simulink model "GesamtsystemAltV2"  (R2018b)
settings: Solver=FixedStepDiscrete  StartTime=0.0  StopTime=1  RelTol=1e-3  EnableMultiTasking=on
libraries: commutil2 x12, c2833xlib x10, c280xlib x8, powerlib_extras x2, simulink x1, c2000lib x1, dspstat3 x1
(part 3 of 3)

== stateflow chart GesamtsystemAltV2/Subsystem/Sortieralgorithmus2 ==
  state setupVariable
    magacin0 = 0;
    magacin1 = 0;
    magacin2 = 0;
    magacin3 = 0;
    magacin4 = 0;
    magacin5 = 0;
    magacin6 = 0;
    magacin0_LastCube = 0;
    magacin1_LastCube = 0;
    magacin2_LastCube = 0;
    magacin3_LastCube = 0;
    magacin4_LastCube = 0;
    magacin5_LastCube = 0;
    magacin6_LastCube = 0;
    magacin = -1;
    cubeCounter = 0;
    blue = 0;
  state wait
  state cubeLoaded
    magacin = -1
  state photoelectricBarrierActivated
  state BlueCube
    entry: blue = blue + 1;
    entry: magacin = findPlaceForBlue();
  state RedCube
    entry: magacin = findPlaceForRed();
  state Black
    magacin = 6;
    entry: magacin6 = magacin6 + 1;
  state DetectedCube
    entry: cubeCounter = cubeCounter +  1;
  setupVariable -> wait : [switchA > 0]
  (default) -> setupVariable
  wait -> cubeLoaded : [after(2,sec)]
  DetectedCube -> cubeLoaded : [movingCube == 0]
  cubeLoaded -> photoelectricBarrierActivated : [(colour < 400) || (colour > 1300)]
  photoelectricBarrierActivated -> BlueCube [order 3] : [((colour >= 1000) && (colour <= 2150)) ]
  photoelectricBarrierActivated -> RedCube [order 2] : [(colour < 1000)]
  photoelectricBarrierActivated -> Black [order 1] : [(colour > 2150) ]
  RedCube -> DetectedCube : [after(1,sec)]
  Black -> DetectedCube : [after(1,sec)]
  BlueCube -> DetectedCube : [after(1,sec)]
  data: magacinOut function_output; magacinOut function_output; colour input; magacin6 local; magacin0_LastCube local; magacin3_LastCube local; magacin2_LastCube local; magacin5_LastCube local; magacin1_LastCube local; magacin6_LastCube local; magacin4_LastCube local; magacin output; magacin0 local; magacin1 local; magacin2 local; magacin3 local; magacin4 local; magacin5 local; movingCube input; cubeCounter local; switchA input; blue local
  function magacinOut  = findPlaceForRed:
    | function magacinOut  = findPlaceForRed
    | 
    | if(magacin1 == 0)
    |             magacinOut = 1;
    |             magacin1 = magacin1 + 1;
    |             magacin1_LastCube = 2;
    |             position = magacin1;
    | elseif (magacin2 == 2 || magacin2 == 3)
    |             magacinOut = 2;
    |             magacin2 = magacin2 + 1; 
    |             magacin2_LastCube = 2;
    |             position = magacin2;
    | elseif (magacin0 < 5)
    |             magacinOut = 0;
    |             magacin0 = magacin0 + 1;
    |             magacin0_LastCube = 2;
    |             position = magacin0;
    | elseif (magacin1 >= 2)
    |             magacinOut = 1;
    |             magacin1 = magacin1 + 1;
    |             magacin1_LastCube = 2;
    |             position = magacin1;  
    | else
    |         if (magacin3 ~= 5)
    |                 magacinOut = 3;
    |                 magacin3 = magacin3 + 1; 
    |                 magacin3_LastCube = 2;
    |                 position = magacin3;
    |         elseif ((magacin1 <= magacin4) && (magacin1 ~= 5))
    |                 magacinOut = 1;
    |                 magacin1 = magacin1 + 1; 
    |                 magacin1_LastCube = 2;
    |                 position = magacin1;
    |         elseif (magacin1 > magacin4)
    |                 magacinOut = 4;
    |                 magacin4 = magacin4 + 1;
    |                 magacin4_lastCube = 2;
    |                 position = magacin4;
    |         elseif ((magacin2 <= magacin5) && (magacin2 ~= 5))
    |                 magacinOut = 2;
    |                 magacin2 = magacin2 + 1;
    |                 magacin2_LastCube = 2;
    |                 position = magacin2;
    |         elseif (magacin2 > magacin5)
    |                 magacinOut = 5;
    |                 magacin5 = magacin5 + 1;
    |                 magacin5_LastCube = 2;
    |                 position = magacin5;
    |         else
    |                 magacinOut = -1;
    |         end            
    | end
  function magacinOut  = findPlaceForBlue:
    | function magacinOut  = findPlaceForBlue
    | 
    | if(magacin2 < 2)  
    |             magacinOut = 2;
    |             magacin2 = (magacin2 + 1);
    |             magacin2_LastCube = 1;
    |             position = magacin2;
    | elseif ((magacin1 == 1) || (magacin1 == 2))
    |             magacinOut = 1;
    |             magacin1 = magacin1 + 1; 
    |             magacin1_LastCube = 1;
    |             position = magacin1;
    | elseif magacin2 == 4
    |             magacinOut = 2;
    |             magacin2 = magacin2 + 1;
    |             magacin2_LastCube = 1;
    |             position = magacin2;
    | elseif magacin0 == 4
    |             magacinOut = 0;
    |             magacin0 = magacin0 + 1;
    |             magacin0_LastCube = 1;
    |             position = magacin0;
    | elseif (magacin3 < 5)
    |             magacinOut = 3;
    |             magacin3 = (magacin3 + 1);
    |             position = magacin3;
    | elseif (magacin4 < 5)
    |             magacinOut = 4;
    |             magacin4 = (magacin4 + 1);
    |             position = magacin4;
    | elseif (magacin5 < 5)
    |             magacinOut = 5;
    |             magacin5 = (magacin5 + 1);
    |             position = magacin5;
    | elseif (blue ~= 22)
    |         if (magacin0 < 5)
    |                 magacinOut = 0;
    |                 magacin0 = (magacin0 + 1);
    |                 position = magacin0;
    |         elseif (magacin1 < 5)
    |                 magacinOut = 1;
    |                 magacin1 = (magacin1 + 1);
    |                 position = magacin1;
    |         elseif (magacin2 < 5)
    |                 magacinOut = 2;
    |                 magacin2 = (magacin2 + 1);
    |                 position = magacin2;
    |         else 
    |                 magacinOut = 6;
    |                 position = magacin6;
    |         end
    | elseif ((magacin0 == 5) && (magacin1 == 5) && (magacin2 == 5) && (magacin3 == 5) && (magacin4 == 5) && (magacin5 == 5))
    |         magacinOut = -1;   
    | else
    |         magacinOut = 6;
    |         position = magacin6;
    | end

== matlab function GesamtsystemAltV2/Subsystem/getAngle2/Messung des absoluten Winkels - Auswertung der Encodersignale/MATLAB Function1 ==
  data: u input; y output; yalt input
function y = fcn(u, yalt)

y = yalt + u;

== matlab function GesamtsystemAltV2/Subsystem/getAngle2/Messung des absoluten Winkels - Auswertung der Encodersignale/MATLAB Function2 ==
  data: u1 input; u1alt input; u2 input; u2alt input; y output; yalt input double; RL output
function [y, RL] = fcn(u1, u1alt, u2, u2alt, yalt)

y = 1;
RL = 1;

if u1alt == 0 && u2alt == 0 && u1 == 0 && u2 == 0
    y = yalt;
end

if u1alt == 0 && u2alt == 0 && u1 == 0 && u2 == 1
    y = 1;
end

if u1alt == 0 && u2alt == 0 && u1 == 1 && u2 == 0
    y = -1;
end

% if u1alt == 0 && u2alt == 0 && u1 == 1 && u2 == 1
%     y = yalt;   % nicht möglich
% end

if u1alt == 0 && u2alt == 1 && u1 == 0 && u2 == 0
    y = -1;
end

if u1alt == 0 && u2alt == 1 && u1 == 0 && u2 == 1
    y = yalt;
end

% if u1alt == 0 && u2alt == 1 && u1 == 1 && u2 == 0
%     y = yalt;   % nicht möglich
% end

if u1alt == 0 && u2alt == 1 && u1 == 1 && u2 == 1
    y = 1;
end

if u1alt == 1 && u2alt == 0 && u1 == 0 && u2 == 0
    y = 1;
end

% if u1alt == 1 && u2alt == 0 && u1 == 0 && u2 == 1
%     y = yalt;   % nicht möglich
% end

if u1alt == 1 && u2alt == 0 && u1 == 1 && u2 == 0
    y = yalt;
end

if u1alt == 1 && u2alt == 0 && u1 == 1 && u2 == 1
    y = -1;
end

% if u1alt == 1 && u2alt == 1 && u1 == 0 && u2 == 0
%     y = yalt;   % nicht möglich
% end

if u1alt == 1 && u2alt == 1 && u1 == 0 && u2 == 1
    y = -1;
end

if u1alt == 1 && u2alt == 1 && u1 == 1 && u2 == 0
    y = 1;
end

if u1alt == 1 && u2alt == 1 && u1 == 1 && u2 == 1
    y = yalt;
end

if y == 1
    RL = 1;
else
    RL = 0;
end

== matlab function GesamtsystemAltV2/Subsystem/getAngle2/Messung des absoluten Winkels - Auswertung der Encodersignale/MATLAB Function3 ==
  data: u input; y output; yalt input
function y = fcn(u, yalt)

y = yalt + u;
